simulink model "OPC_UA_Test_Daniel"  (R2024b)
settings: Solver=VariableStepDiscrete  StartTime=0.0  StopTime=inf  MaxStep=0.01  RelTol=1e-3
libraries: opcualib x1
settings Model: Creator=Are-Laptop  LastModifiedBy=Are-Laptop

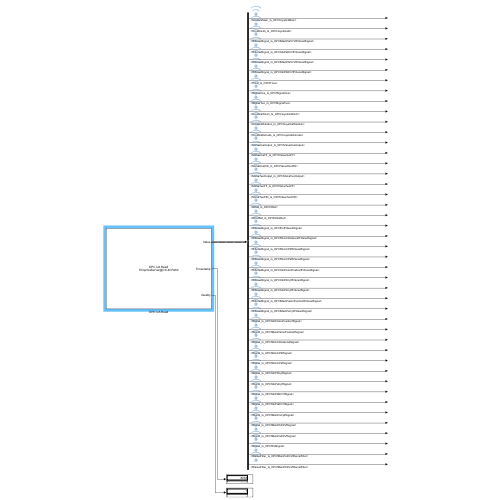
[thumbnail: Simulink's stored preview of the top-level diagram]
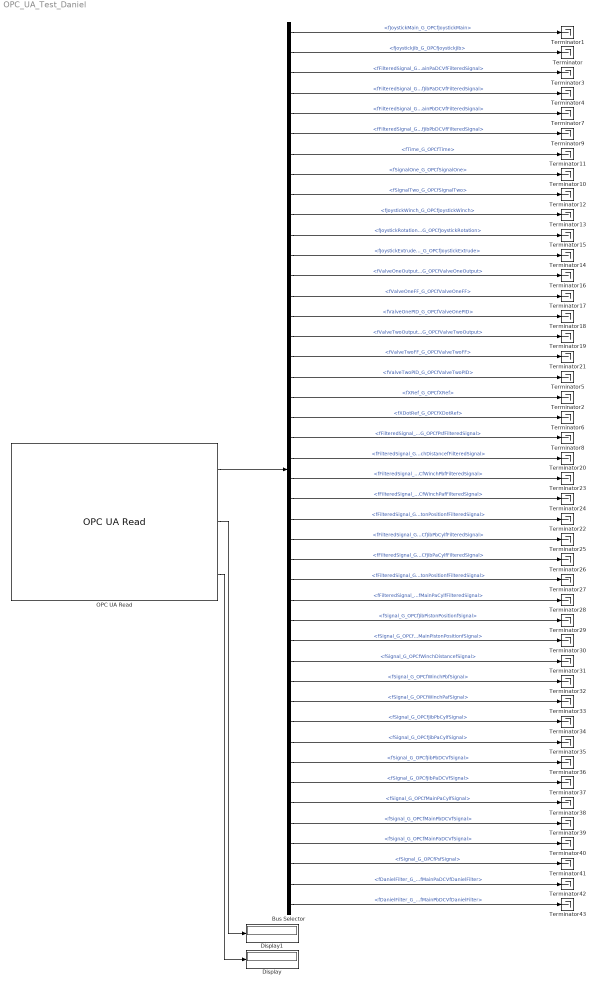
== system OPC_UA_Test_Daniel ==
  Bus Selector : BusSelector  OutputSignals=fJoystickMain_G_OPCfJoystickMain,fJoystickJib_G_OPCfJoystickJib,fFilteredSignal_G_OPCfMainPaDCVfFilteredSignal,fFilteredSignal_G_OPCfJibPaDCVfFilteredSignal,fFilteredSignal_G_OPCfMainPbDCVfFilteredSignal,fFilteredSignal_G_OPCfJibPbDCVfFilteredSignal,fTime_G_OPCfTime,fSignalOne_G_OPCfSignalOne,fSignalTwo_G_OPCfSignalTwo,fJoystickWinch_G_OPCfJoystickWinch,fJoystickRotation_G_OPCfJoystickRotation,fJoystickExtrude_G_OPCfJoystickExtrude,fValveOneOutput_G_OPCfValveOneOutput,fValveOneFF_G_OPCfValveOneFF,fValveOnePID_G_OPCfValveOnePID,fValveTwoOutput_G_OPCfValveTwoOutput,fValveTwoFF_G_OPCfValveTwoFF,fValveTwoPID_G_OPCfValveTwoPID,fXRef_G_OPCfXRef,fXDotRef_G_OPCfXDotRef,fFilteredSignal_G_OPCfPsfFilteredSignal,fFilteredSignal_G_OPCfWinchDistancefFilteredSignal,fFilteredSignal_G_OPCfWinchPbfFilteredSignal,fFilteredSignal_G_OPCfWinchPafFilteredSignal,fFilteredSignal_G_OPCfJibPistonPositionfFilteredSignal,fFilteredSignal_G_OPCfJibPbCylfFilteredSignal,fFilteredSignal_G_OPCfJibPaCylfFilteredSignal,fFilteredSignal_G_OPCfMainPistonPositionfFilteredSignal,fFilteredSignal_G_OPCfMainPaCylfFilteredSignal,fSignal_G_OPCfJibPistonPositionfSignal,fSignal_G_OPCfMainPistonPositionfSignal,fSignal_G_OPCfWinchDistancefSignal,fSignal_G_OPCfWinchPbfSignal,fSignal_G_OPCfWinchPafSignal,fSignal_G_OPCfJibPbCylfSignal,fSignal_G_OPCfJibPaCylfSignal,fSignal_G_OPCfJibPbDCVfSignal,fSignal_G_OPCfJibPaDCVfSignal,fSignal_G_OPCfMainPaCylfSignal,fSignal_G_OPCfMainPbDCVfSignal,fSignal_G_OPCfMainPaDCVfSignal,fSignal_G_OPCfPsfSignal,fDanielFilter_G_OPCfMainPaDCVfDanielFilter,fDanielFilter_G_OPCfMainPbDCVfDanielFilter
  Display : Display
  Display1 : Display
  OPC UA Read : opcualib/OPC UA Read  SelectedServer=TcOpcUaServer@CX-4CFA60  ServerList=TcOpcUaServer@CX-4CFA60  NodeList={ '1', 'fTime', '4', 'G_OPC.fTime', '0'; '2', 'fSignalOne', '4', 'G_OPC.fSignalOne', '0'; '3', 'fSignalTwo', '4', 'G_OPC.fSignalTwo', '0'; '4', 'fJoystickWinch', '4', 'G_OPC.fJoystickWinch', '0'; '5', 'fJoystickRotation', '4', 'G_OPC.fJoystickRotation', '0'; '6', 'fJoystickMain', '4', 'G_OPC.fJoystickMain', '0'; '7', 'fJoystickJib', '4', 'G_OPC.fJoystickJib', '0'; '8', 'fJoystickExtrude', '4', 'G_OPC.fJoystickExtrude', '0'; '9', 'fValveOneOutput', '4', 'G_OPC.fValveOneOutput', '0'; '10', 'fValveOneFF', '4', 'G_OPC.fValveOneFF', '0'; '11', 'fValveOnePID', '4', 'G_OPC.fValveOnePID', '0'; '12', 'fValveTwoOutput', '4', 'G_OPC.fValveTwoOutput', '0'; '13', 'fValveTwoFF', '4', 'G_OPC.fValveTwoFF', '0'; '14', 'fValveTwoPID', '4', 'G_OPC.fValveTwoPID', '0'; '15', 'fXRef', '4', 'G_OPC.fXRef', '0'; '16', 'fXDotRef', '4', 'G_OPC.fXDotRef', '0'; '17', 'fSignal', '4', 'G_OPC.fPs.fSignal', '0'; '18', 'fFilteredSignal', '4', 'G_OPC.fPs.fFilteredSignal', '0'; '19', 'fSignal', '4', 'G_OPC.fWinchDistance.fSignal', '0'; '20', 'fFilteredSignal', '4', 'G_OPC.fWinchDistance.fFilteredSignal', '0'; '21', 'fSignal', '4', 'G_OPC.fWinchPb.fSignal', '0'; '22', 'fFilteredSignal', '4', 'G_OPC.fWinchPb.fFilteredSignal', '0'; '23', 'fSignal', '4', 'G_OPC.fWinchPa.fSignal', '0'; '24', 'fFilteredSignal', '4', 'G_OPC.fWinchPa.fFilteredSignal', '0'; '25', 'fSignal', '4', 'G_OPC.fJibPistonPosition.fSignal', '0'; '26', 'fFilteredSignal', '4', 'G_OPC.fJibPistonPosition.fFilteredSignal', '0'; '27', 'fSignal', '4', 'G_OPC.fJibPbCyl.fSignal', '0'; '28', 'fFilteredSignal', '4', 'G_OPC.fJibPbCyl.fFilteredSignal', '0'; '29', 'fSignal', '4', 'G_OPC.fJibPaCyl.fSignal', '0'; '30', 'fFilteredSignal', '4', 'G_OPC.fJibPaCyl.fFilteredSignal', '0'; '31', 'fSignal', '4', 'G_OPC.fJibPbDCV.fSignal', '0'; '32', 'fFilteredSignal', '4', 'G_OPC.fJibPbDCV.fFilteredSignal', '0'; '33', 'fSignal', '4', 'G_OPC.fJibPaDCV.fSignal', '0'; '34', 'fFilteredSignal', '4', 'G_OPC.fJibPaDCV.fFilteredSignal', '0'; '35', 'fSignal', '4', 'G_OPC.fMainPistonPosition.fSignal', '0'; '36', 'fFilteredSignal', '4', 'G_OPC.fMainPistonPosition.fFilteredSignal', '0'; '37', 'fSignal', '4', 'G_OPC.fMainPaCyl.fSignal', '0'; '38', 'fFilteredSignal', '4', 'G_OPC.fMainPaCyl.fFilteredSignal', '0'; '39', 'fSignal', '4', 'G_OPC.fMainPbDCV.fSignal', '0'; '40', 'fFilteredSignal', '4', 'G_OPC.fMainPbDCV.fFilteredSignal', '0'; '41', 'fSignal', '4', 'G_OPC.fMainPaDCV.fSignal', '0'; '42', 'fFilteredSignal', '4', 'G_OPC.fMainPaDCV.fFilteredSignal', '0'; '43', 'fDanielFilter', '4', 'G_OPC.fMainPaDCV.fDanielFilter', '0'; '44', 'fDanielFilter', '4', 'G_OPC.fMainPbDCV.fDanielFilter', '0' }  ShowQualityPort=on  ShowTimestampPort=on  ShowTimestampPortAs=Seconds since start  SampleTime=-1
  Terminator{,1..43} (44 alike) : Terminator
  wires:
  OPC UA Read/1 -> Bus Selector/1
  OPC UA Read/3 -> Display/1
  Bus Selector/31 -> Terminator30/1  "<fSignal_G_OPCfMainPistonPositionfSignal>"
  OPC UA Read/2 -> Display1/1
  Bus Selector/40 -> Terminator39/1  "<fSignal_G_OPCfMainPbDCVfSignal>"
  Bus Selector/2 -> Terminator/1  "<fJoystickJib_G_OPCfJoystickJib>"
  Bus Selector/42 -> Terminator41/1  "<fSignal_G_OPCfPsfSignal>"
  Bus Selector/38 -> Terminator37/1  "<fSignal_G_OPCfJibPaDCVfSignal>"
  Bus Selector/1 -> Terminator1/1  "<fJoystickMain_G_OPCfJoystickMain>"
  Bus Selector/9 -> Terminator12/1  "<fSignalTwo_G_OPCfSignalTwo>"
  Bus Selector/7 -> Terminator11/1  "<fTime_G_OPCfTime>"
  Bus Selector/3 -> Terminator3/1  "<fFilteredSignal_G_OPCfMainPaDCVfFilteredSignal>"
  Bus Selector/5 -> Terminator7/1  "<fFilteredSignal_G_OPCfMainPbDCVfFilteredSignal>"
  Bus Selector/10 -> Terminator13/1  "<fJoystickWinch_G_OPCfJoystickWinch>"
  Bus Selector/8 -> Terminator10/1  "<fSignalOne_G_OPCfSignalOne>"
  Bus Selector/6 -> Terminator9/1  "<fFilteredSignal_G_OPCfJibPbDCVfFilteredSignal>"
  Bus Selector/4 -> Terminator4/1  "<fFilteredSignal_G_OPCfJibPaDCVfFilteredSignal>"
  Bus Selector/13 -> Terminator16/1  "<fValveOneOutput_G_OPCfValveOneOutput>"
  Bus Selector/11 -> Terminator15/1  "<fJoystickRotation_G_OPCfJoystickRotation>"
  Bus Selector/12 -> Terminator14/1  "<fJoystickExtrude_G_OPCfJoystickExtrude>"
  Bus Selector/14 -> Terminator17/1  "<fValveOneFF_G_OPCfValveOneFF>"
  Bus Selector/15 -> Terminator18/1  "<fValveOnePID_G_OPCfValveOnePID>"
  Bus Selector/16 -> Terminator19/1  "<fValveTwoOutput_G_OPCfValveTwoOutput>"
  Bus Selector/21 -> Terminator8/1  "<fFilteredSignal_G_OPCfPsfFilteredSignal>"
  Bus Selector/19 -> Terminator2/1  "<fXRef_G_OPCfXRef>"
  Bus Selector/17 -> Terminator21/1  "<fValveTwoFF_G_OPCfValveTwoFF>"
  Bus Selector/20 -> Terminator6/1  "<fXDotRef_G_OPCfXDotRef>"
  Bus Selector/18 -> Terminator5/1  "<fValveTwoPID_G_OPCfValveTwoPID>"
  Bus Selector/28 -> Terminator27/1  "<fFilteredSignal_G_OPCfMainPistonPositionfFilteredSignal>"
  Bus Selector/26 -> Terminator25/1  "<fFilteredSignal_G_OPCfJibPbCylfFilteredSignal>"
  Bus Selector/24 -> Terminator24/1  "<fFilteredSignal_G_OPCfWinchPafFilteredSignal>"
  Bus Selector/22 -> Terminator20/1  "<fFilteredSignal_G_OPCfWinchDistancefFilteredSignal>"
  Bus Selector/29 -> Terminator28/1  "<fFilteredSignal_G_OPCfMainPaCylfFilteredSignal>"
  Bus Selector/27 -> Terminator26/1  "<fFilteredSignal_G_OPCfJibPaCylfFilteredSignal>"
  Bus Selector/25 -> Terminator22/1  "<fFilteredSignal_G_OPCfJibPistonPositionfFilteredSignal>"
  Bus Selector/23 -> Terminator23/1  "<fFilteredSignal_G_OPCfWinchPbfFilteredSignal>"
  Bus Selector/30 -> Terminator29/1  "<fSignal_G_OPCfJibPistonPositionfSignal>"
  Bus Selector/32 -> Terminator31/1  "<fSignal_G_OPCfWinchDistancefSignal>"
  Bus Selector/33 -> Terminator32/1  "<fSignal_G_OPCfWinchPbfSignal>"
  Bus Selector/34 -> Terminator33/1  "<fSignal_G_OPCfWinchPafSignal>"
  Bus Selector/35 -> Terminator34/1  "<fSignal_G_OPCfJibPbCylfSignal>"
  Bus Selector/36 -> Terminator35/1  "<fSignal_G_OPCfJibPaCylfSignal>"
  Bus Selector/41 -> Terminator40/1  "<fSignal_G_OPCfMainPaDCVfSignal>"
  Bus Selector/37 -> Terminator36/1  "<fSignal_G_OPCfJibPbDCVfSignal>"
  Bus Selector/39 -> Terminator38/1  "<fSignal_G_OPCfMainPaCylfSignal>"
  Bus Selector/43 -> Terminator42/1  "<fDanielFilter_G_OPCfMainPaDCVfDanielFilter>"
  Bus Selector/44 -> Terminator43/1  "<fDanielFilter_G_OPCfMainPbDCVfDanielFilter>"
